simulink model "test_verifier"  (R2021b)
settings: Solver=FixedStepDiscrete  StartTime=0.0  StopTime=10.0  FixedStep=0.10000000000000001  RelTol=1e-3  EnableMultiTasking=on
undefined symbols (not defined in the file): m, n, sldvsubsys
libraries: sldvlib x3, hdlsllib x2, simulink x1
settings Model: Creator=mattiabacci  LastModifiedBy=Alessandro
settings SolverCC: AlgebraicLoopSolver=TrustRegion  AutoInsertRateTranBlk=on
settings DataIOCC: SaveOutput=off  DSMLogging=off  SaveTime=off  SignalLoggingName=logsout_Validator
settings OptimizationCC: LifeSpan=inf
settings DebuggingCC: InheritedTsInSrcMsg=none  AllowSymbolicDim=off  SFUnexpectedBacktrackingDiag=warning  SFNoUnconditionalDefaultTransitionDiag=warning  SFExecutionAtInitializationDiag=none  ArithmeticOperatorsInVariantConditions=warning
settings ModelReferenceCC: UpdateModelReferenceTargets=IfOutOfDate
settings SFSimCC: SimUseLocalCustomCode=off  CustomCodeUndefinedFunction=UseInterfaceOnly
settings RTWCC: RTWUseLocalCustomCode=off
settings CodeAppCC: StateflowObjectComments=on
settings GRTTargetCC: TargetLangStandard=C89/C90 (ANSI)
settings ConfigComp: CovEnable=on  RecordCoverage=on  CovSaveName=coveragedata  CovMetricSettings=owe  CovEnableCumulative=off  CovSaveCumulativeToWorkspaceVar=on  CovSaveSingleToWorkspaceVar=on  CovOutputDir=sldv_covoutput/test_verifier  CovModelRefEnable=on  CovSFcnEnable=off  DVMode=PropertyProving  DVTestSuiteOptimization=Auto  DVDetectOutOfBounds=on  DVModelReferenceHarness=on

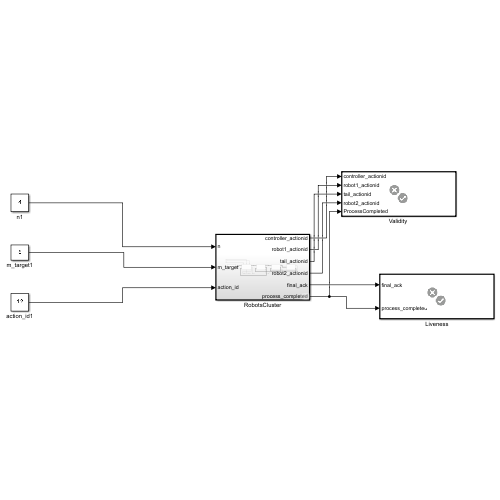
[thumbnail: Simulink's stored preview of the top-level diagram]
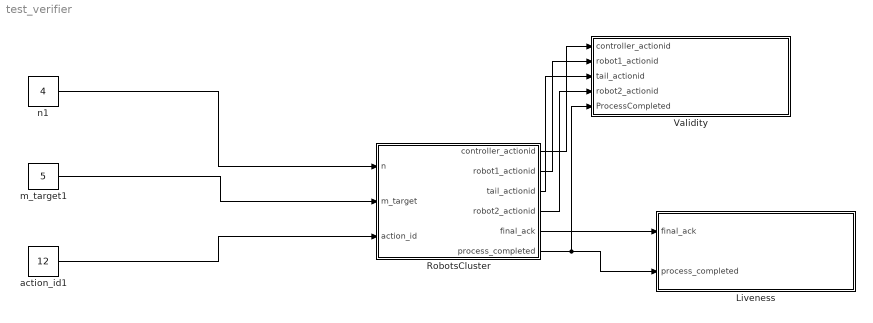
== system test_verifier ==
  Liveness : Subsystem  Tag=VerificationSubsystem  DisableCoverage=on  LoadFcn=sldvsubsys('check')  TreatAsAtomicUnit=on  SimViewingDevice=on  mask(VerificationSubsystem){}
      mask init:
      | sldvsubsys('maskInit');
      settings: CopyFcn=sldvsubsys('copy');  OpenFcn=open_system(gcb,'force');
      settings: PreSaveFcn=|
      | set_param(gcb,'SimViewingDevice','on');
      | sldvsubsys('check');
      mask Help: helpview(fullfile(docroot,'toolbox','sldv','sldv.map'),'verificationsubsystem')
      mask Display: image(imread('sldvicon_versubsys.png','BackGroundColor',[1 1 1]),'center');
  RobotsCluster : Subsystem  TreatAsAtomicUnit=on
  "Validity " : Subsystem  Tag=VerificationSubsystem  DisableCoverage=on  LoadFcn=sldvsubsys('check')  TreatAsAtomicUnit=on  SimViewingDevice=on  mask(VerificationSubsystem){}
      mask init:
      | sldvsubsys('maskInit');
      settings: CopyFcn=sldvsubsys('copy');  OpenFcn=open_system(gcb,'force');
      settings: PreSaveFcn=|
      | set_param(gcb,'SimViewingDevice','on');
      | sldvsubsys('check');
      mask Help: helpview(fullfile(docroot,'toolbox','sldv','sldv.map'),'verificationsubsystem')
      mask Display: image(imread('sldvicon_versubsys.png','BackGroundColor',[1 1 1]),'center');
  action_id1 : Constant  Value=12  VectorParams1D=off  OutDataTypeStr=double
  m_target1 : Constant  Value=5  VectorParams1D=off  OutDataTypeStr=double
  n1 : Constant  Value=4  VectorParams1D=off  OutDataTypeStr=double
  wires:
  n1/1 -> RobotsCluster/1(n)
  action_id1/1 -> RobotsCluster/3(action_id)
  RobotsCluster/6(process_completed) -> "Validity "/5(ProcessCompleted), Liveness/2(process_completed)
  m_target1/1 -> RobotsCluster/2(m_target)
  RobotsCluster/5(final_ack) -> Liveness/1(final_ack)
  RobotsCluster/1(controller_actionid) -> "Validity "/1(controller_actionid)
  RobotsCluster/2(robot1_actionid) -> "Validity "/2(robot1_actionid)
  RobotsCluster/3(tail_actionid) -> "Validity "/3(tail_actionid)
  RobotsCluster/4(robot2_actionid) -> "Validity "/4(robot2_actionid)

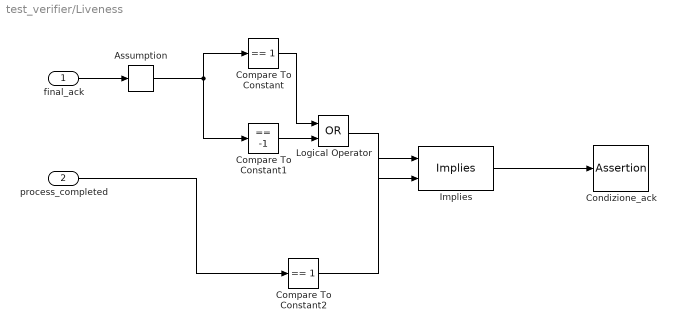
== system test_verifier/Liveness ==
  final_ack : Inport  OutDataTypeStr=double
  process_completed : Inport  Port=2  OutDataTypeStr=double
  Assumption : sldvlib/Objectives and Constraints/Assumption  enabled=off  customAVTBlockType=Assumption  intervals={-1,1}  initial=off  dispValues=on  outEnabled=on
      settings: AttributesFormatString=%<intervals>  SourceProductBaseCode=SL
  Compare To Constant : hdlsllib/Logic and Bit Operations/Compare To Constant  relop===  const=1  OutDataTypeStr=boolean
      settings: SourceProductBaseCode=SL
  Compare To Constant1 : hdlsllib/Logic and Bit Operations/Compare To Constant  relop===  const=-1  OutDataTypeStr=boolean
      settings: SourceProductBaseCode=SL
  Compare To Constant2 : simulink/Logic and Bit Operations/Compare To Constant  relop===  const=1  OutDataTypeStr=boolean
  Condizione_ack : Assertion  StopWhenAssertionFail=off
  Implies : sldvlib/Verification Utilities/Implies
      settings: SourceProductBaseCode=SL
  Logical Operator : Logic  Operator=OR  AllPortsSameDT=off  OutDataTypeStr=boolean
  wires:
  final_ack/1 -> Assumption/1
  process_completed/1 -> Compare To Constant2/1
  Compare To Constant2/1 -> Implies/1
  Implies/1 -> Condizione_ack/1
  Assumption/1 -> Compare To Constant1/1, Compare To Constant/1
  Compare To Constant/1 -> Logical Operator/1
  Compare To Constant1/1 -> Logical Operator/2
  Logical Operator/1 -> Implies/2

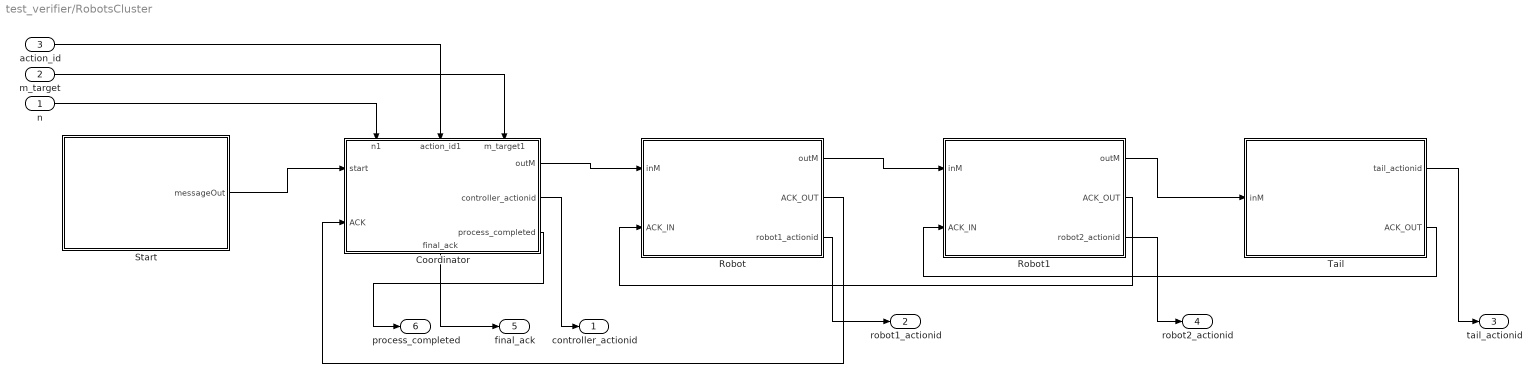
== system test_verifier/RobotsCluster ==
  n : Inport  OutDataTypeStr=double
  m_target : Inport  Port=2  OutDataTypeStr=double
  action_id : Inport  Port=3  OutDataTypeStr=double
  Coordinator : Stateflow chart  TreatAsAtomicUnit=on
      settings: PortSchema="{\"entries\":[{\"content\":{\"sides\":[{\"content\":{\"connectorIds\":[\"In4\",\"In5\"]},\"type\":\"ConnectorPlacement.EquallySpacedRectSide\",\"uuid\":\"25a90162-2ba2-405c-92ca-476f1557c0bb\"},{\"content\":{\"connectorIds\":[\"Out2\",\"Out3\",\"Out4\"],\"side\":\"RIGHT\"},\"type\":\"ConnectorPlacement.EquallySpacedRectSide\",\"uuid\":\"ea2c754e-f922-41fb-9e01-83d1994128b8\"},{\"content\":{\"connectorIds\":[\"In1\",\"In2\",\"In3\"],\"side\":\"TOP\"},\"type\":\"ConnectorPlacement.EquallySpacedRectSide\",\"uuid\":\"d29a44b1-123a-44b5-acd5-1d638e11f489\"},{\"content\":{\"connectorIds\":[\"Out1\"],\"side\":\"BOTTOM\"},\"type\":\"ConnectorPlacement.EquallySpacedRectSide\",\"uuid\":\"db450b56-4665-4bcd-8d5b-e9c3289a225c\"}]},\"type\":\"ConnectorPlacement.EquallySpacedConnector\",\"uuid\":\"f4e25f01-003d-4860-be41-4fe0a0784bf6\"}],\"packageUris\":[\"http://schema.mathworks.com/mf0/Connector/R2020b\"],\"version\":\"1.0\"}"
  Robot : Stateflow chart  TreatAsAtomicUnit=on
  Robot1 : Stateflow chart  TreatAsAtomicUnit=on
  Start : Stateflow chart  TreatAsAtomicUnit=on
  Tail : Stateflow chart  TreatAsAtomicUnit=on
  controller_actionid : Outport
  robot1_actionid : Outport  Port=2
  tail_actionid : Outport  Port=3
  robot2_actionid : Outport  Port=4
  final_ack : Outport  Port=5  OutDataTypeStr=double
  process_completed : Outport  Port=6  OutDataTypeStr=double
  wires:
  Start/1(messageOut) -> Coordinator/4(start)
  Robot/2(ACK_OUT) -> Coordinator/5(ACK)
  Coordinator/2(outM) -> Robot/1(inM)
  action_id/1 -> Coordinator/2(action_id1)
  n/1 -> Coordinator/1(n1)
  m_target/1 -> Coordinator/3(m_target1)
  Coordinator/3(controller_actionid) -> controller_actionid/1
  Robot/3(robot1_actionid) -> robot1_actionid/1
  Tail/1(tail_actionid) -> tail_actionid/1
  Robot1/2(ACK_OUT) -> Robot/2(ACK_IN)
  Robot/1(outM) -> Robot1/1(inM)
  Robot1/1(outM) -> Tail/1(inM)
  Robot1/3(robot2_actionid) -> robot2_actionid/1
  Coordinator/1(final_ack) -> final_ack/1
  Tail/2(ACK_OUT) -> Robot1/2(ACK_IN)
  Coordinator/4(process_completed) -> process_completed/1

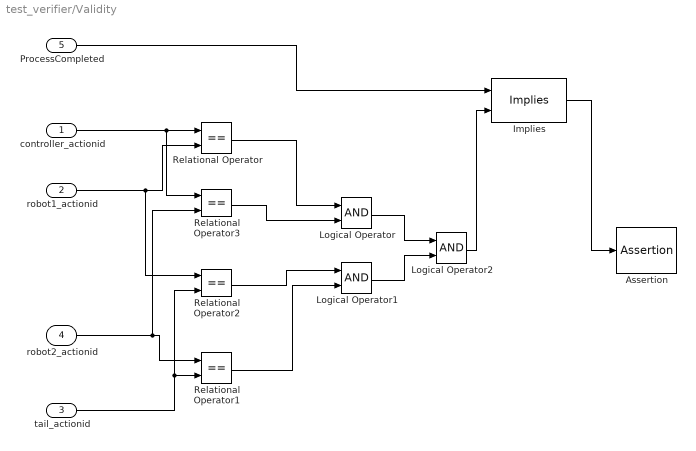
== system test_verifier/Validity  ==
  controller_actionid : Inport
  robot1_actionid : Inport  Port=2
  tail_actionid : Inport  Port=3
  robot2_actionid : Inport  Port=4
  ProcessCompleted : Inport  Port=5
  Assertion : Assertion  StopWhenAssertionFail=off
  Implies : sldvlib/Verification Utilities/Implies
      settings: SourceProductBaseCode=SL
  Logical Operator : Logic  AllPortsSameDT=off  OutDataTypeStr=boolean
  Logical Operator1 : Logic  AllPortsSameDT=off  OutDataTypeStr=boolean
  Logical Operator2 : Logic  AllPortsSameDT=off  OutDataTypeStr=boolean
  Relational Operator{,1..3} (4 alike) : RelationalOperator  Operator===  OutDataTypeStr=boolean  RndMeth=Simplest
  wires:
  controller_actionid/1 -> Relational Operator3/1, Relational Operator/1
  robot1_actionid/1 -> Relational Operator2/1, Relational Operator/2
  robot2_actionid/1 -> Relational Operator3/2, Relational Operator1/1
  tail_actionid/1 -> Relational Operator2/2, Relational Operator1/2
  Relational Operator/1 -> Logical Operator/1
  Relational Operator3/1 -> Logical Operator/2
  Relational Operator2/1 -> Logical Operator1/1
  Relational Operator1/1 -> Logical Operator1/2
  Logical Operator/1 -> Logical Operator2/1
  Logical Operator1/1 -> Logical Operator2/2
  Logical Operator2/1 -> Implies/2
  ProcessCompleted/1 -> Implies/1
  Implies/1 -> Assertion/1

== stateflow chart test_verifier/RobotsCluster/Robot ==
  state Begin
    entry:
    flag=0
  state Decision
    entry:
    m_now= inM.data(1);
    m_target= inM.data(2);
    n= inM.data(3);
    action_id = inM.data(4)
    robot1_actionid = action_id;
    randN = Random();
    if randN > 0
    m_now = m_now + 1;
    end
  state ACK
    entry:
    ACK_OUT.data = ACK_IN.data;
    send(ACK_OUT);
  state OutputInterface
    entry:
    if m_now==m_target
    ACK_OUT.data = 1;
    send(ACK_OUT);
    else
    out=[0,m_target, n,action_id];
    out(1) = m_now;
    outM.data=out;
    send(outM);
    end
  (default) -> Begin
  Begin -> Decision [order 1] : inM
  OutputInterface -> Begin
  ACK -> Begin
  Begin -> ACK [order 2] : ACK_IN
  Decision -> OutputInterface
  data: r function_output; m_now local; m_target local; n local; out local; randN local; outM output size=[1 4]; flag local; inM input size=4; ACK_IN input; ACK_OUT output; action_id local; robot1_actionid output
  function r = Random:
    | function r = Random
    | %#codegen
    | r = rand(1);
    | end

== stateflow chart test_verifier/RobotsCluster/Robot1 ==
  state Begin
    entry:
    flag=0
  state Decision
    entry:
    m_now= inM.data(1);
    m_target= inM.data(2);
    n= inM.data(3);
    action_id = inM.data(4)
    robot2_actionid = action_id;
    randN = Random();
    if randN > 0
    m_now = m_now + 1;
    end
  state ACK
    entry:
    ACK_OUT.data = ACK_IN.data;
    send(ACK_OUT);
  state OutputInterface
    entry:
    if m_now==m_target
    ACK_OUT.data = 1;
    send(ACK_OUT);
    else
    out=[0,m_target, n,action_id];
    out(1) = m_now;
    outM.data=out;
    send(outM);
    end
  (default) -> Begin
  Begin -> Decision [order 1] : inM
  OutputInterface -> Begin
  ACK -> Begin
  Begin -> ACK [order 2] : ACK_IN
  Decision -> OutputInterface
  data: r function_output; m_now local; m_target local; n local; out local; randN local; outM output size=[1 4]; flag local; inM input size=4; ACK_IN input; ACK_OUT output; action_id local; robot2_actionid output
  function r = Random:
    | function r = Random
    | %#codegen
    | r = rand(1);
    | end

== stateflow chart test_verifier/RobotsCluster/Start ==
  state Begin
    entry:
    messageOut.data = 1;
    send(messageOut);
  (default) -> Begin
  data: messageOut output

== stateflow chart test_verifier/RobotsCluster/Tail ==
  state Decision
    entry:
    m_now= inM.data(1);
    m_target= inM.data(2);
    n= inM.data(3);
    randN = Random();
    tail_actionid = inM.data(4);
    if randN > 0.5
    m_now = m_now + 1;
    end
  state Begin
    entry:
    flag=0
  state OutputInterface
    entry:
    if m_now>m_target
    ACK_OUT.data = 1;
    send(ACK_OUT);
    else
    ACK_OUT.data = -1;
    send(ACK_OUT);
    end
  (default) -> Begin
  Begin -> Decision : inM
  OutputInterface -> Begin
  Decision -> OutputInterface
  data: r function_output; tail_actionid output; m_now local; m_target local; n local; randN local; flag local; inM input size=[1 4]; ACK_OUT output
  function r = Random:
    | function r = Random
    | %#codegen
    | r = rand(1);
    | end

== stateflow chart test_verifier/RobotsCluster/Coordinator ==
  state Begin
    entry:
  state Decision
    entry:
    randN = Random();
    out=[0,m_target, n,action_id];
    controller_actionid = action_id;
    if randN > 0.5
    m_now = m_now + 1;
    end
    out(1) = m_now;
    outM.data=out;
    send(outM);
  state ACK
    entry:
    ackValue= ACK.data;
  state Final_state
    entry:
    final_ack = ackValue;
    process_completed = 1;
  (default) -> Begin : {m_now=0,
      | m_target=m_target1,
      | n=n1
      | action_id=action_id1}
  Begin -> Decision [order 1] : start
  Decision -> Begin
  Begin -> ACK [order 2] : ACK
  ACK -> Final_state : [ackValue==-1 ||ackValue==1]
  data: r function_output; final_ack output; n1 input; action_id1 input; m_target1 input; start input; randN local; m_now local; n local; m_target local; flag local; out local; outM output size=[1 4]; ACK input; ackValue local; action_id local; controller_actionid output; process_completed output
  function r = Random:
    | function r = Random
    | %#codegen
    | r = rand(1);
    | end
